simulink library "dspstat3"  (Simulink 6.0)
settings: Solver=ode45  SolverMode=SingleTasking  StartTime=0.0  StopTime=10.0  RelTol=1e-3
values from neighbouring files (symbols this model uses):
  D = D + B    [rebuffer_delay.m]
undefined symbols (not defined in the file or in its folder): Rows
libraries: dspsigattribs x7, simulink x3, dspmtrx3 x2, dspsrcs4 x1, dspindex x1, dspstat3 x1
settings Model: RequirementInfo=9  CovMetricSettings=d  Creator=szlotkin  LastModifiedBy=mlongfri  ExtModeAutoUpdateStatusClock=off  ProdHWDeviceType=Specified
settings DataIOCC: SignalLoggingName=logsOut
settings OptimizationCC: BooleanDataType=off
settings DebuggingCC: CheckExecutionContextPreStartOutputMsg=on  CheckExecutionContextRuntimeOutputMsg=on  SolverPrmCheckMsg=none
settings HardwareCC: ProdHWDeviceType=Specified  TargetUnknown=on
settings SFSimCC: SFSimApplyToAllLibs=on  SFSimBuildMode=Incremental

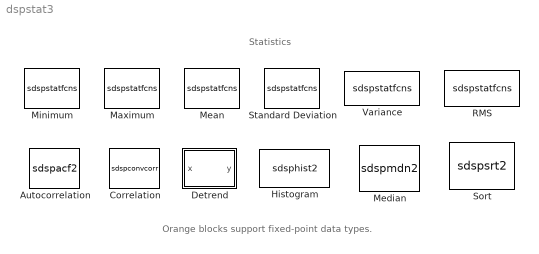
== system dspstat3 ==
  note: Statistics
  note: Orange blocks support fixed-point data types.
  Autocorrelation : S-Function  DialogController=dspDDGCreate  DialogControllerArgs=DataTag0  FunctionName=sdspacf2  Parameters=AllPositiveLags,maxlag,bias,domain,dtInfo.prodOutputMode,dtInfo.prodOutputWordLength,dtInfo.prodOutputFracLength,dtInfo.accumMode,dtInfo.accumWordLength,dtInfo.accumFracLength,dtInfo.outputMode,dtInfo.outputWordLength,dtInfo.outputFracLength,dtInfo.roundingMode,dtInfo.overflowMode  mask(Autocorrelation){AllPositiveLags=on, maxlag=1, bias=None, domain=Time, additionalParams=off, allowOverrides=on, outputMode=Same as accumulator, outputWordLength=16, outputFracLength=15, accumMode=Inherit via internal rule, accumWordLength=32, accumFracLength=30, prodOutputMode=Inherit via internal rule, prodOutputWordLength=32, prodOutputFracLength=30, roundingMode=Floor, overflowMode=off, LockScale=off}
      mask prompts: AllPositiveLags "Compute all non-negative lags"; maxlag "Maximum non-negative lag (less than input length):"; bias "Scaling:"; domain "Computation domain:"; additionalParams "--------------- Show additional parameters ---------------"; allowOverrides "Allow overrides from DSP Fixed-Point Attributes blocks"; outputMode "Fixed-point output attributes:"; outputWordLength "Output word length:"; outputFracLength "Output fraction length:"; accumMode "Fixed-point accumulator attributes:"; accumWordLength "Accumulator word length:"; accumFracLength "Accumulator fraction length:"; prodOutputMode "Fixed-point product output attributes:"; prodOutputWordLength "Product output word length:"; prodOutputFracLength "Product output fraction length:"; roundingMode "Round integer calculations toward:"; overflowMode "Saturate on integer overflow"; LockScale "Lock scaling"
      mask help:
      | Compute the autocorrelation of vectors or frame-based matrices. For frame-based inputs, the block computes along the input's columns.
      |
      | When "Compute all non-negative lags" is selected, it computes using lags in the range [0, length(input)-1]. Otherwise, it computes using lags in the range [0, maxLag], where you specify the value of maxLag in the "Maximum non-negative lag" parameter.
      mask init:
      | dtInfo = dspblkacf2('init');
      settings: CopyFcn=dspfixptcopycallback
      mask Help: web(dspbhelp);
      mask StyleString: checkbox,edit,popup(None|Biased|Unbiased|Unity at zero-lag),popup(Time|Frequency),checkbox,checkbox,popup(Same as accumulator|Same as product output|Same as input|Binary point scaling|Slope and bias scaling|User-defined),edit,edit,popup(Inherit via internal rule|Same as product output|Same as input|Binary point scaling|Slope and bias scaling|User-defined),edit,edit,popup(Inherit via internal rule|Same as input|Binary point scaling|Slope and bias scaling|User-defined),edit,edit,popup(Floor|Nearest),checkbox,checkbox
      mask Display: disp('ACF')
  Correlation : S-Function  DialogController=dspDDGCreate  DialogControllerArgs=DataTag1  FunctionName=sdspconvcorr  Parameters=domain,1,dtInfo.prodOutputMode,dtInfo.prodOutputWordLength,dtInfo.prodOutputFracLength,dtInfo.accumMode,dtInfo.accumWordLength,dtInfo.accumFracLength,dtInfo.outputMode,dtInfo.outputWordLength,dtInfo.outputFracLength,dtInfo.roundingMode,dtInfo.overflowMode  mask(Correlation){domain=Time, additionalParams=off, allowOverrides=on, outputMode=Same as accumulator, outputWordLength=16, outputFracLength=15, accumMode=Inherit via internal rule, accumWordLength=32, accumFracLength=30, prodOutputMode=Inherit via internal rule, prodOutputWordLength=32, prodOutputFracLength=30, roundingMode=Floor, overflowMode=off, LockScale=off}
      mask prompts: domain "Computation domain:"; additionalParams "------- Show additional parameters -------"; allowOverrides "Allow overrides from DSP Fixed-Point Attributes blocks"; outputMode "Fixed-point output attributes:"; outputWordLength "Output word length:"; outputFracLength "Output fraction length:"; accumMode "Fixed-point accumulator attributes:"; accumWordLength "Accumulator word length:"; accumFracLength "Accumulator fraction length:"; prodOutputMode "Fixed-point product output attributes:"; prodOutputWordLength "Product output word length:"; prodOutputFracLength "Product output fraction length:"; roundingMode "Round integer calculations toward:"; overflowMode "Saturate on integer overflow"; LockScale "Lock scaling"
      mask help: Correlate two inputs. The block computes in the time domain or frequency domain. To minimize the number of computations, select "Fastest" in the Computation domain parameter. To minimize memory use, select "Time" in the Computation domain parameter.
      mask init:
      | dtInfo = dspblkconvcorr('init');
      settings: CopyFcn=dspfixptcopycallback
      mask Help: web(dspbhelp);
      mask StyleString: popup(Time|Frequency|Fastest),checkbox,checkbox,popup(Same as accumulator|Same as product output|Same as first input|Binary point scaling|Slope and bias scaling|User-defined),edit,edit,popup(Inherit via internal rule|Same as product output|Same as first input|Binary point scaling|Slope and bias scaling|User-defined),edit,edit,popup(Inherit via internal rule|Same as first input|Binary point scaling|Slope and bias scaling|User-defined),edit,edit,popup(Floor|Nearest),checkbox,checkbox
      mask Display: disp('XCORR')
  Detrend : Subsystem  PropExecContextAcrossSSBoundary=on
      mask Type: Detrend
      mask Description: Remove linear trend from vector input.
      mask Help: web(dspbhelp);
      mask Display: plot(0,0,100,100,[12 20 24 32 38 44 49 54 67 69 71 78 81 89],[56 76 60 79 75 83 80 87 65 76 84 86 91 89],[],[],[],[],[],[],[12 20 24 32 38 44 49 54 67 69 71 78 81 89],[12 31 13 31 27 34 30 36 13 23 30 31 34 32],[4 96],[61 90],[47 47 42 47 52],[64 44 50 44 50],[4 96],[23 23])
  Histogram : S-Function  DialogController=dspDDGCreate  DialogControllerArgs=DataTag5  FunctionName=sdsphist2  Parameters=umin,umax,nbins,normalized,run,reset,trigtype,dtInfo.prodOutputMode,dtInfo.prodOutputWordLength,dtInfo.prodOutputFracLength,dtInfo.accumMode,dtInfo.accumWordLength,dtInfo.accumFracLength,dtInfo.roundingMode,dtInfo.overflowMode  mask(Histogram){umin=0, umax=10, nbins=11, normalized=off, run=off, reset=on, trigtype=Non-zero sample, additionalParams=off, allowOverrides=on, accumMode=Same as input, accumWordLength=32, accumFracLength=30, prodOutputMode=Same as input, prodOutputWordLength=32, prodOutputFracLength=30, roundingMode=Floor, overflowMode=off}
      mask prompts: umin "Minimum value of input:"; umax "Maximum  value of input:"; nbins "Number of bins:"; run "Running histogram"; reset "Reset port"; trigtype "Trigger type:"; additionalParams "--------------- Show additional parameters ---------------"; allowOverrides "Allow overrides from DSP Attributes blocks"; accumMode "Fixed-point accumulator attributes"; accumWordLength "Accumulator word length:"; accumFracLength "Accumulator fraction length:"; prodOutputMode "Fixed-point product output attributes:"; prodOutputWordLength "Product output word length:"; prodOutputFracLength "Product output fraction length:"; roundingMode "Round integer calculations toward:"; overflowMode "Saturate on integer overflow"
      mask help:
      | Histogram of the vector elements.  If running histogram is selected, block returns the histogram of the input elements over time.
      |
      | The accumulator and product output parameters are only used for complex fixed-point inputs.
      mask init:
      | [s,x,y] = dspblkhist2('icon');
      | dtInfo = dspblkhist2('init');
      | trigtype=trigtype-1;
      settings: CopyFcn=dspfixptcopycallback
      mask Help: web(dspbhelp);
      mask StyleString: edit,edit,edit,checkbox,checkbox,checkbox,popup(None|Rising edge|Falling edge|Either edge|Non-zero sample),checkbox,checkbox,popup(Same as product output|Same as input|Binary point scaling|Slope and bias scaling|User-defined),edit,edit,popup(Same as input|Binary point scaling|Slope and bias scaling|User-defined),edit,edit,popup(Floor|Nearest),checkbox
      mask Display:
      | plot(x,y);
      | port_label('input',s.i1,s.i1s);
      | port_label('input',s.i2,s.i2s);
  Maximum : S-Function  DialogController=dspDDGCreate  DialogControllerArgs=DataTag6  FunctionName=sdspstatfcns  Parameters=statfcn,fcn,reset,dtInfo.prodOutputMode,dtInfo.prodOutputWordLength,dtInfo.prodOutputFracLength,dtInfo.accumMode,dtInfo.accumWordLength,dtInfo.accumFracLength,0,0,0,dtInfo.roundingMode,dtInfo.overflowMode  mask(Maximum){fcn=Value and Index, reset=None, additionalParams=off, allowOverrides=on, accumMode=Same as product output, accumWordLength=32, accumFracLength=30, prodOutputMode=Same as input, prodOutputWordLength=32, prodOutputFracLength=30, roundingMode=Floor, overflowMode=off, LockScale=off}
      mask prompts: fcn "Mode:"; reset "Reset port:"; additionalParams "--------------- Show additional parameters ---------------"; allowOverrides "Allow overrides from DSP Attributes blocks"; accumMode "Fixed-point accumulator attributes:"; accumWordLength "Accumulator word length:"; accumFracLength "Accumulator fraction length:"; prodOutputMode "Fixed-point product output attributes:"; prodOutputWordLength "Product output word length:"; prodOutputFracLength "Product output fraction length:"; roundingMode "Round integer calculations toward:"; overflowMode "Saturate on integer overflow"; LockScale "Lock scaling"
      mask help:
      | Value and/or index of maximum element in vector. If "Running" is selected for the Mode parameter, the block returns the maximum of the input elements over time.
      |
      | The accumulator and product output parameters are only used for complex fixed-point inputs.
      mask init:
      | [s, x, y] = dspblkminmax('icon','max');
      | reset=reset-1;
      | statfcn=5;map = [0 2 3 1];
      | fcn = map(fcn);
      | dtInfo = dspblkminmax('init');
      settings: CopyFcn=dspfixptcopycallback
      mask Help: web(dspbhelp);
      mask StyleString: popup(Value and Index|Value|Index|Running),popup(None|Rising edge|Falling edge|Either edge|Non-zero sample),checkbox,checkbox,popup(Same as product output|Same as input|Binary point scaling|Slope and bias scaling|User-defined),edit,edit,popup(Same as input|Binary point scaling|Slope and bias scaling|User-defined),edit,edit,popup(Floor|Nearest),checkbox,checkbox
      mask Display:
      | plot(x,y);
      | port_label('input',s.i1,s.i1s);
      | port_label('input',s.i2,s.i2s);
      | port_label('output',s.o1,s.o1s);
      | port_label('output',s.o2,s.o2s);
  Mean : S-Function  DialogController=dspDDGCreate  DialogControllerArgs=DataTag7  FunctionName=sdspstatfcns  Parameters=fcn,run,reset,0,0,0,dtInfo.accumMode,dtInfo.accumWordLength,dtInfo.accumFracLength,dtInfo.outputMode,dtInfo.outputWordLength,dtInfo.outputFracLength,dtInfo.roundingMode,dtInfo.overflowMode  mask(Mean){run=off, reset_popup=None, additionalParams=off, allowOverrides=on, outputMode=Same as accumulator, outputWordLength=32, outputFracLength=30, accumMode=Same as input, accumWordLength=32, accumFracLength=30, roundingMode=Floor, overflowMode=off, LockScale=off}
      mask prompts: run "Running mean"; reset_popup "Reset port"; additionalParams "--------------- Show additional parameters ---------------"; allowOverrides "Allow overrides from DSP Attributes blocks"; outputMode "Fixed-point output attributes:"; outputWordLength "Output word length:"; outputFracLength "Output fraction length:"; accumMode "Fixed-point accumulator attributes"; accumWordLength "Accumulator word length:"; accumFracLength "Accumulator fraction length:"; roundingMode "Round integer calculations toward:"; overflowMode "Saturate on integer overflow"; LockScale "Lock scaling"
      mask help: Mean of the vector elements. If "Running mean" is selected, the block returns the mean of the input elements over time.
      mask init:
      | [s,x,y] = dspblkmean2('icon');
      | reset=reset_popup-1;
      | fcn=3;
      | dtInfo = dspblkmean2('init');
      settings: CopyFcn=dspfixptcopycallback
      mask Help: web(dspbhelp);
      mask StyleString: checkbox,popup(None|Rising edge|Falling edge|Either edge|Non-zero sample),checkbox,checkbox,popup(Same as accumulator|Same as input|Binary point scaling|Slope and bias scaling|User-defined),edit,edit,popup(Same as input|Binary point scaling|Slope and bias scaling|User-defined),edit,edit,popup(Floor|Nearest),checkbox,checkbox
      mask Display:
      | plot(x,y);
      | port_label('input',s.i1,s.i1s);
      | port_label('input',s.i2,s.i2s);
  Median : S-Function  DialogController=dspDDGCreate  DialogControllerArgs=DataTag8  FunctionName=sdspmdn2  Parameters=sortAlg,dtInfo.prodOutputMode,dtInfo.prodOutputWordLength,dtInfo.prodOutputFracLength,dtInfo.accumMode,dtInfo.accumWordLength,dtInfo.accumFracLength,dtInfo.outputMode,dtInfo.outputWordLength,dtInfo.outputFracLength,dtInfo.roundingMode,dtInfo.overflowMode  mask(Median){sortAlg=Quick sort, additionalParams=off, allowOverrides=off, outputMode=Same as accumulator, outputWordLength=16, outputFracLength=15, accumMode=Same as product output, accumWordLength=32, accumFracLength=30, prodOutputMode=Same as input, prodOutputWordLength=32, prodOutputFracLength=30, roundingMode=Floor, overflowMode=off, LockScale=off}
      mask prompts: sortAlg "Sort algorithm:"; additionalParams "--------------- Show additional parameters ---------------"; allowOverrides "Allow overrides from DSP Attributes blocks"; outputMode "Fixed-point output attributes:"; outputWordLength "Output word length:"; outputFracLength "Output fraction length:"; accumMode "Fixed-point accumulator attributes"; accumWordLength "Accumulator word length:"; accumFracLength "Accumulator fraction length:"; prodOutputMode "Fixed-point product output attributes:"; prodOutputWordLength "Product output word length:"; prodOutputFracLength "Product output fraction length:"; roundingMode "Round integer calculations toward:"; overflowMode "Saturate on integer overflow"; LockScale "Lock scaling"
      mask help:
      | Median value of input elements.
      |
      | The accumulator and product output parameters are only used for complex fixed-point inputs.
      mask init:
      | [x,y] = dspblkmedian('icon');
      | dtInfo = dspblkmedian('init');
      settings: CopyFcn=dspfixptcopycallback
      mask Help: web(dspbhelp);
      mask StyleString: popup(Quick sort|Insertion sort),checkbox,checkbox,popup(Same as accumulator|Same as product output|Same as input|Binary point scaling|Slope and bias scaling|User-defined),edit,edit,popup(Same as product output|Same as input|Binary point scaling|Slope and bias scaling|User-defined),edit,edit,popup(Same as input|Binary point scaling|Slope and bias scaling|User-defined),edit,edit,popup(Floor|Nearest),checkbox,checkbox
      mask Display: plot(x,y);
  Minimum : S-Function  DialogController=dspDDGCreate  DialogControllerArgs=DataTag9  FunctionName=sdspstatfcns  Parameters=statfcn,fcn,reset,dtInfo.prodOutputMode,dtInfo.prodOutputWordLength,dtInfo.prodOutputFracLength,dtInfo.accumMode,dtInfo.accumWordLength,dtInfo.accumFracLength,0,0,0,dtInfo.roundingMode,dtInfo.overflowMode  mask(Minimum){fcn=Value and Index, reset=None, additionalParams=off, allowOverrides=on, accumMode=Same as product output, accumWordLength=32, accumFracLength=30, prodOutputMode=Same as input, prodOutputWordLength=32, prodOutputFracLength=30, roundingMode=Floor, overflowMode=off, LockScale=off}
      mask prompts: fcn "Mode:"; reset "Reset port"; additionalParams "--------------- Show additional parameters ---------------"; allowOverrides "Allow overrides from DSP Attributes blocks"; accumMode "Fixed-point accumulator attributes:"; accumWordLength "Accumulator word length:"; accumFracLength "Accumulator fraction length:"; prodOutputMode "Fixed-point product output attributes:"; prodOutputWordLength "Product output word length:"; prodOutputFracLength "Product output fraction length:"; roundingMode "Round integer calculations toward:"; overflowMode "Saturate on integer overflow"; LockScale "Lock scaling"
      mask help:
      | Value and/or index of minimum element in vector. If "Running" is selected for the Mode parameter, the block returns the minimum of the input elements over time.
      |
      | The accumulator and product output parameters are only used for complex fixed-point inputs.
      mask init:
      | [s, x, y] = dspblkminmax('icon','min');
      | reset=reset-1;
      | statfcn=4;map = [0 2 3 1];
      | fcn = map(fcn);
      | dtInfo = dspblkminmax('init');
      settings: CopyFcn=dspfixptcopycallback
      mask Help: web(dspbhelp);
      mask StyleString: popup(Value and Index|Value|Index|Running),popup(None|Rising edge|Falling edge|Either edge|Non-zero sample),checkbox,checkbox,popup(Same as input|Same as product output|Binary point scaling|Slope and bias scaling|User-defined),edit,edit,popup(Same as input|Binary point scaling|Slope and bias scaling|User-defined),edit,edit,popup(Floor|Nearest),checkbox,checkbox
      mask Display:
      | plot(x,y);
      | port_label('input',s.i1,s.i1s);
      | port_label('input',s.i2,s.i2s);
      | port_label('output',s.o1,s.o1s);
      | port_label('output',s.o2,s.o2s);
  RMS : S-Function  FunctionName=sdspstatfcns  Parameters=fcn,run,reset  mask(RMS){run=off, reset_popup=None}
      mask prompts: run "Running RMS"; reset_popup "Reset port"
      mask help: Root-mean-square of the vector elements. If "Running RMS" is selected, the block returns the RMS of the input elements over time.
      mask init:
      | [s,x] = dspblkrms2('icon');
      | fcn=2;
      | reset=reset_popup-1;
      mask Help: web(dspbhelp);
      mask StyleString: checkbox,popup(None|Rising edge|Falling edge|Either edge|Non-zero sample)
      mask CallbackString: dspblkrms2;|
      mask Display:
      | disp(x);
      | port_label('input',s.i1,s.i1s);
      | port_label('input',s.i2,s.i2s);
  Sort : S-Function  DialogController=dspDDGCreate  DialogControllerArgs=DataTag10  FunctionName=sdspsrt2  Parameters=dir,otype,sortAlg,dtInfo.prodOutputMode,dtInfo.prodOutputWordLength,dtInfo.prodOutputFracLength,dtInfo.accumMode,dtInfo.accumWordLength,dtInfo.accumFracLength,dtInfo.roundingMode,dtInfo.overflowMode  mask(Sort){otype=Value and Index, dir=Ascending, sortAlg=Quick sort, additionalParams=off, allowOverrides=on, accumMode=Same as product output, accumWordLength=32, accumFracLength=30, prodOutputMode=Same as input, prodOutputWordLength=32, prodOutputFracLength=30, roundingMode=Floor, overflowMode=off}
      mask prompts: otype "Mode:"; dir "Sort order:"; sortAlg "Sort algorithm:"; additionalParams "--------------- Show additional parameters ---------------"; allowOverrides "Allow overrides from DSP Attributes blocks"; accumMode "Fixed-point accumulator attributes"; accumWordLength "Accumulator word length:"; accumFracLength "Accumulator fraction length:"; prodOutputMode "Fixed-point product output attributes:"; prodOutputWordLength "Product output word length:"; prodOutputFracLength "Product output fraction length:"; roundingMode "Round integer calculations toward:"; overflowMode "Saturate on integer overflow"
      mask help:
      | Value and/or index of sorted elements in vector or matrix.  For matrix inputs, the elements are sorted columnwise.
      |
      | The accumulator and product output parameters are only used for complex fixed-point inputs.
      mask init:
      | [s,x,y] = dspblksort('icon',dir,otype);
      | dtInfo = dspblksort('init');
      settings: CopyFcn=dspfixptcopycallback
      mask Help: web(dspbhelp);
      mask StyleString: popup(Value and Index|Value|Index),popup(Ascending|Descending),popup(Quick sort|Insertion sort),checkbox,checkbox,popup(Same as product output|Same as input|Binary point scaling|Slope and bias scaling|User-defined),edit,edit,popup(Same as input|Binary point scaling|Slope and bias scaling|User-defined),edit,edit,popup(Floor|Nearest),checkbox
      mask Display:
      | plot(x,y);
      | port_label('input',s.i1,s.i1s);
      | port_label('input',s.i2,s.i2s);
      | port_label('output',s.o1,s.o1s);
      | port_label('output',s.o2,s.o2s);
  Standard Deviation : S-Function  FunctionName=sdspstatfcns  Parameters=fcn,run,reset  mask(Standard Deviation){run=off, reset_popup=None}
      mask prompts: run "Running standard deviation"; reset_popup "Reset port"
      mask help: Standard deviation of the vector elements. If "Running standard deviation" is selected, the block returns the standard deviation of the input elements over time.
      mask init:
      | [s,x,y] = dspblkstd2('icon');
      | fcn=1;
      |  %Set the flag to compute the standard deviation
      | reset=reset_popup-1;
      mask Help: web(dspbhelp);
      mask StyleString: checkbox,popup(None|Rising edge|Falling edge|Either edge|Non-zero sample)
      mask CallbackString: dspblkstd2;|
      mask Display:
      | plot(x,y);
      | port_label('input',s.i1,s.i1s);
      | port_label('input',s.i2,s.i2s);
  Variance : S-Function  DialogController=dspDDGCreate  DialogControllerArgs=DataTag11  FunctionName=sdspstatfcns  Parameters=fcn,run,reset,dtInfo.prodOutputMode,dtInfo.prodOutputWordLength,dtInfo.prodOutputFracLength,dtInfo.accumMode,dtInfo.accumWordLength,dtInfo.accumFracLength,dtInfo.outputMode,dtInfo.outputWordLength,dtInfo.outputFracLength,dtInfo.roundingMode,dtInfo.overflowMode  mask(Variance){run=off, reset_popup=None, additionalParams=off, allowOverrides=on, outputMode=Same as accumulator, outputWordLength=32, outputFracLength=30, accumMode=Same as product output, accumWordLength=32, accumFracLength=30, prodOutputMode=Same as input, prodOutputWordLength=32, prodOutputFracLength=30, roundingMode=Floor, overflowMode=off, LockScale=off}
      mask prompts: run "Running variance"; reset_popup "Reset port"; additionalParams "--------------- Show additional parameters ---------------"; allowOverrides "Allow overrides from DSP Attributes blocks"; outputMode "Fixed-point output attributes:"; outputWordLength "Output word length:"; outputFracLength "Output fraction length:"; accumMode "Fixed-point accumulator attributes"; accumWordLength "Accumulator word length:"; accumFracLength "Accumulator fraction length:"; prodOutputMode "Fixed-point product output attributes:"; prodOutputWordLength "Product output word length:"; prodOutputFracLength "Product output fraction length:"; roundingMode "Round integer calculations toward:"; overflowMode "Saturate on integer overflow"; LockScale "Lock scaling"
      mask help: Variance of the vector elements. If "Running variance" is selected, the block returns the variance of the input elements over time.
      mask init:
      | [s,x] = dspblkvar2('icon');
      | fcn=0; %Set the flag to compute the variance
      | reset=reset_popup-1;
      | dtInfo = dspblkvar2('init');
      settings: CopyFcn=dspfixptcopycallback
      mask Help: web(dspbhelp);
      mask StyleString: checkbox,popup(None|Rising edge|Falling edge|Either edge|Non-zero sample),checkbox,checkbox,popup(Same as accumulator|Same as product output|Same as input|Binary point scaling|Slope and bias scaling|User-defined),edit,edit,popup(Same as input|Same as product output|Binary point scaling|Slope and bias scaling|User-defined),edit,edit,popup(Same as input|Binary point scaling|Slope and bias scaling|User-defined),edit,edit,popup(Floor|Nearest),checkbox,checkbox
      mask Display:
      | disp(x);
      | port_label('input',s.i1,s.i1s);
      | port_label('input',s.i2,s.i2s);

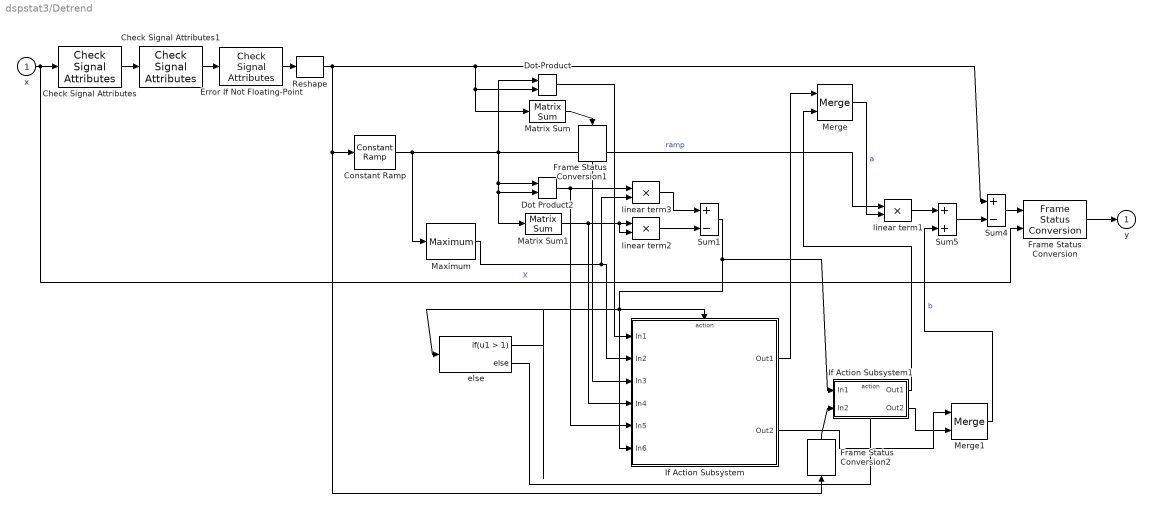
== system dspstat3/Detrend ==
  x : Inport  LatchInput=off
  Check Signal Attributes : dspsigattribs/Check Signal Attributes  SigAttribCheckMethod=Does not match attributes exactly  Complexity=Ignore  Frame=Ignore  DimsCheckMethod=Is...  Dimensions=Vector (1-D or 2-D) or scalar  DatatypeCheckMethod=Ignore  DatatypeGeneral=Boolean  DtypeFloatSpecific=Any floating-point  DtypeFixedSpecific=Any fixed-point  DtypeIntSpecific=Any integer  SampleMode=Ignore
  Check Signal Attributes1 : dspsigattribs/Check Signal Attributes  SigAttribCheckMethod=Matches attributes exactly  Complexity=Ignore  Frame=Frame-based  DimsCheckMethod=Is...  Dimensions=Row vector (2-D)  DatatypeCheckMethod=Ignore  DatatypeGeneral=Boolean  DtypeFloatSpecific=Any floating-point  DtypeFixedSpecific=Any fixed-point  DtypeIntSpecific=Any integer  SampleMode=Ignore
  Constant Ramp : dspsrcs4/Constant Ramp  L=Rows  Slope=1  dataType=Same as input  isSigned=on  wordLen=16  udDataType=sfix(16)  fracBitsMode=Best precision  numFracBits=15  Offset=1
  Dot Product : simulink/Math Operations/Dot Product  OutDataType=sfix(16)  OutScaling=2^-10  DoSatur=off
  Dot Product2 : simulink/Math Operations/Dot Product  OutDataType=sfix(16)  OutScaling=2^-10  DoSatur=off
  Error If Not Floating-Point : dspsigattribs/Check Signal Attributes  SigAttribCheckMethod=Does not match attributes exactly  Complexity=Ignore  Frame=Ignore  DimsCheckMethod=Ignore  Dimensions=1-D  DatatypeCheckMethod=Is...  DatatypeGeneral=Floating-point  DtypeFloatSpecific=Any floating-point  DtypeFixedSpecific=Any fixed-point  DtypeIntSpecific=Any integer  SampleMode=Ignore
  Frame Status Conversion : dspsigattribs/Frame Status Conversion  growRefPort=on  outframe=Frame-based
  Frame Status Conversion1 : dspsigattribs/Frame Status Conversion  Orientation=down  growRefPort=off  outframe=Sample-based
  Frame Status Conversion2 : dspsigattribs/Frame Status Conversion  Orientation=up  growRefPort=off  outframe=Sample-based
  If Action Subsystem : Subsystem  TreatAsAtomicUnit=on  PropExecContextAcrossSSBoundary=on
  If Action Subsystem1 : Subsystem  TreatAsAtomicUnit=on  PropExecContextAcrossSSBoundary=on
  Matrix Sum : dspmtrx3/Matrix Sum  DialogController=dspDDGCreate  DialogControllerArgs=DataTag2  Dim=Columns  roundingMode=Floor  overflowMode=off
  Matrix Sum1 : dspmtrx3/Matrix Sum  DialogController=dspDDGCreate  DialogControllerArgs=DataTag3  Dim=Columns  roundingMode=Floor  overflowMode=off
  Maximum : dspstat3/Maximum  DialogController=dspDDGCreate  DialogControllerArgs=DataTag4  fcn=Value  reset=None  roundingMode=Floor  overflowMode=off
  Merge : Merge
  Merge1 : Merge
  Reshape : simulink/Math Operations/Reshape  OutputDimensionality=Column vector  OutputDimensions=[1,1]
  Sum1 : Sum  Inputs=+-  SaturateOnIntegerOverflow=on  InputSameDT=on
  Sum4 : Sum  Inputs=+-  SaturateOnIntegerOverflow=on  InputSameDT=on
  Sum5 : Sum  Inputs=2  SaturateOnIntegerOverflow=on  InputSameDT=on
  else : If  IfExpression=u1 > 1  ZeroCross=off
  linear term1 : Product  SaturateOnIntegerOverflow=on  InputSameDT=on
  linear term2 : Product  SaturateOnIntegerOverflow=on  InputSameDT=on
  linear term3 : Product  SaturateOnIntegerOverflow=on  InputSameDT=on
  y : Outport  InitialOutput=0
  wires:
  x/1 -> Check Signal Attributes/1, Frame Status Conversion/2  "X"
  Merge/1 -> linear term1/2  "a"
  linear term1/1 -> Sum5/1
  Merge1/1 -> Sum5/2  "b"
  Sum5/1 -> Sum4/2
  Dot Product2/1 -> linear term3/1, If Action Subsystem/5(In5)
  Matrix Sum1/1 -> If Action Subsystem/4(In4), linear term2/1, linear term2/2
  Maximum/1 -> linear term3/2, If Action Subsystem/2(In2)
  Check Signal Attributes/1 -> Check Signal Attributes1/1
  Reshape/1 -> Matrix Sum/1, Dot Product/2, Sum4/1, Constant Ramp/1, Frame Status Conversion2/1
  Check Signal Attributes1/1 -> Error If Not Floating-Point/1
  Sum4/1 -> Frame Status Conversion/1
  Frame Status Conversion/1 -> y/1
  Constant Ramp/1 -> Dot Product2/2, Matrix Sum1/1, Dot Product2/1, linear term1/1, Dot Product/1, Maximum/1  "ramp"
  else/1 -> If Action Subsystem/Action
  linear term3/1 -> Sum1/1
  linear term2/1 -> Sum1/2
  Dot Product/1 -> If Action Subsystem/1(In1)
  Matrix Sum/1 -> Frame Status Conversion1/1
  Sum1/1 -> If Action Subsystem1/1(In1), If Action Subsystem/6(In6), else/1
  If Action Subsystem/1(Out1) -> Merge/1
  If Action Subsystem1/2(Out2) -> Merge1/2
  If Action Subsystem/2(Out2) -> Merge1/1
  else/2 -> If Action Subsystem1/Action
  Frame Status Conversion1/1 -> If Action Subsystem/3(In3)
  Frame Status Conversion2/1 -> If Action Subsystem1/2(In2)
  If Action Subsystem1/1(Out1) -> Merge/2
  Error If Not Floating-Point/1 -> Reshape/1

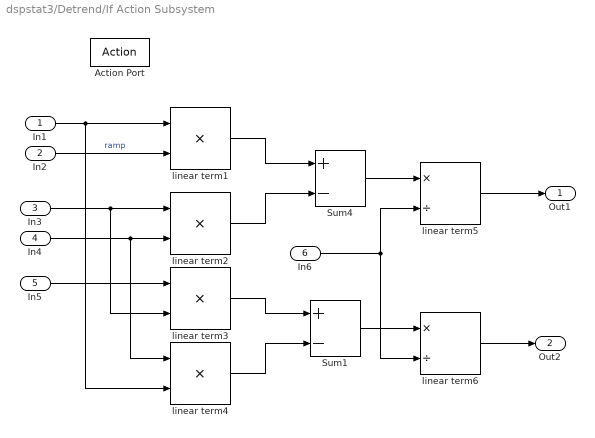
== system dspstat3/Detrend/If Action Subsystem ==
  In1 : Inport  LatchInput=off
  In2 : Inport  Port=2  LatchInput=off
  In3 : Inport  Port=3  LatchInput=off
  In4 : Inport  Port=4  LatchInput=off
  In5 : Inport  Port=5  LatchInput=off
  In6 : Inport  Port=6  LatchInput=off
  Action Port : ActionPort
  Sum1 : Sum  Inputs=+-  SaturateOnIntegerOverflow=on  InputSameDT=on
  Sum4 : Sum  Inputs=+-  SaturateOnIntegerOverflow=on  InputSameDT=on
  linear term{1..4} (4 alike) : Product  SaturateOnIntegerOverflow=on  InputSameDT=on
  linear term5 : Product  Inputs=*/  SaturateOnIntegerOverflow=on  InputSameDT=on
  linear term6 : Product  Inputs=*/  SaturateOnIntegerOverflow=on  InputSameDT=on
  Out1 : Outport
  Out2 : Outport  Port=2
  wires:
  In1/1 -> linear term1/1, linear term4/2
  In2/1 -> linear term1/2  "ramp"
  In3/1 -> linear term2/1, linear term3/2
  In4/1 -> linear term2/2, linear term4/1
  linear term1/1 -> Sum4/1
  linear term2/1 -> Sum4/2
  linear term3/1 -> Sum1/1
  linear term4/1 -> Sum1/2
  In6/1 -> linear term5/2, linear term6/2
  Sum4/1 -> linear term5/1
  Sum1/1 -> linear term6/1
  In5/1 -> linear term3/1
  linear term5/1 -> Out1/1
  linear term6/1 -> Out2/1

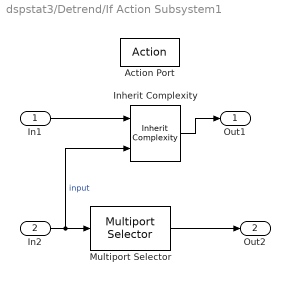
== system dspstat3/Detrend/If Action Subsystem1 ==
  In1 : Inport  LatchInput=off
  In2 : Inport  Port=2  LatchInput=off
  Action Port : ActionPort
  Inherit Complexity : dspsigattribs/Inherit Complexity
  Multiport Selector : dspindex/Multiport Selector  rowsOrCols=Rows  idxCellArray=1  idxErrMode=Clip Index
  Out1 : Outport
  Out2 : Outport  Port=2
  wires:
  In2/1 -> Multiport Selector/1, Inherit Complexity/2  "input"
  Multiport Selector/1 -> Out2/1
  In1/1 -> Inherit Complexity/1
  Inherit Complexity/1 -> Out1/1
